simulink model "zaibotongbu_lulonghao"  (Simulink 6.0)
settings: Solver=ode3  StartTime=0.0  StopTime=10.0  FixedStep=0.000001  RelTol=1e-3
libraries: dsparch4 x2, commchan2 x1, dspswit3 x1, commsynccomp2 x1
settings Model: LastModifiedBy=xxgcxy602

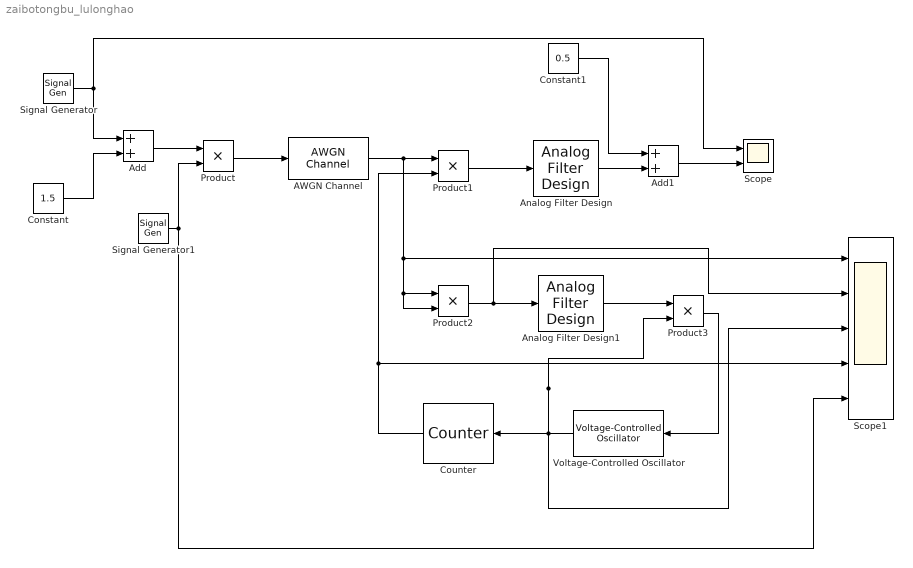
== system zaibotongbu_lulonghao ==
  AWGN Channel : commchan2/AWGN Channel  seed=0  noiseMode=Variance from mask  EbNodB=10  EsNodB=10  SNRdB=10  bitsPerSym=1  Ps=1  Tsym=1  variance=0.01
  Add : Sum  OutScaling=2^-10
  Add1 : Sum  OutScaling=2^-10
  Analog Filter Design : dsparch4/Analog Filter Design  method=Butterworth  filttype=Lowpass  N=8  Wlo=2*pi*1000  Whi=80  Rp=2  Rs=40
  Analog Filter Design1 : dsparch4/Analog Filter Design  method=Butterworth  filttype=Bandpass  N=8  Wlo=2*pi*19000  Whi=2*pi*21000  Rp=2  Rs=40
  Constant : Constant  Value=1.5
  Constant1 : Constant  Value=0.5
  Counter : dspswit3/Counter  Orientation=left  Direction=Up  CountEvent=Rising edge  CounterSize=User defined  MaxCount=1  InitialCount=0  Output=Count  HitValue=32  ResetInput=off  SamplesPerFrame=1  Ts=1  CntDtype=single  HitDtype=Logical
  Product{,1..3} (4 alike) : Product  RndMeth=Zero
  Scope : Scope  NumInputPorts=2
      settings: YMin=-1~-5  YMax=1~5
  Scope1 : Scope  NumInputPorts=5
      settings: YMin=-5~0~-5~-5~-5  YMax=5~17.5~5~5~5
  Signal Generator : SignalGenerator  Frequency=1000
  Signal Generator1 : SignalGenerator  Amplitude=1.5  Frequency=10000
  Voltage-Controlled Oscillator : commsynccomp2/Voltage-Controlled Oscillator  Orientation=left  Ac=1  Fc=20300  Kc=4000  Ph=0
  wires:
  Constant/1 -> Add/2
  Add/1 -> Product/1
  Product/1 -> AWGN Channel/1
  Voltage-Controlled Oscillator/1 -> Counter/1, Product3/2, Scope1/3
  AWGN Channel/1 -> Product1/1, Product2/1, Product2/2, Scope1/1
  Product2/1 -> Analog Filter Design1/1, Scope1/2
  Product1/1 -> Analog Filter Design/1
  Analog Filter Design/1 -> Add1/2
  Constant1/1 -> Add1/1
  Add1/1 -> Scope/2
  Signal Generator/1 -> Add/1, Scope/1
  Analog Filter Design1/1 -> Product3/1
  Product3/1 -> Voltage-Controlled Oscillator/1
  Counter/1 -> Product1/2, Scope1/4
  Signal Generator1/1 -> Product/2, Scope1/5
